simulink model "virtual_v11"  (R2022a)
settings: Solver=VariableStepAuto  StartTime=0.0  StopTime=50  RelTol=1e-3
libraries: slpidlib x5
settings Model: Creator=leona  LastModifiedBy=leona

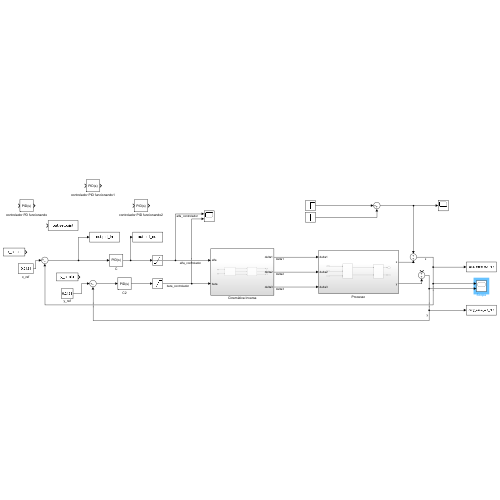
[thumbnail: Simulink's stored preview of the top-level diagram]
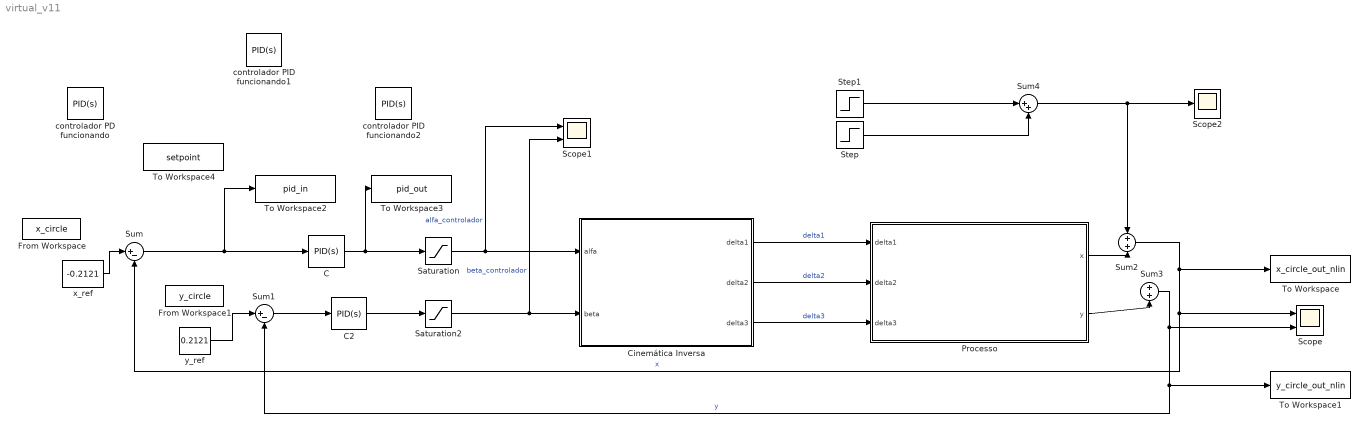
== system virtual_v11 ==
  C : slpidlib/PID Controller  Controller=PID  Form=Parallel  TimeDomain=Continuous-time  UseExternalTs=off  SampleTime=-1  IntegratorMethod=Forward Euler  FilterMethod=Forward Euler  ControllerParametersSource=internal  P=-0.3  I=-0.05  UseKiTs=off  D=-0.45  N=100  UseFilter=on  TunerSelectOption=Transfer Function Based (PID Tuner App)  InitialConditionSource=internal  InitialConditionForIntegrator=0  InitialConditionForFilter=0  DifferentiatorICPrevScaledInput=0  ExternalReset=none  TrackingMode=off  Kt=1  LimitOutput=off  SatLimitsSource=internal  UpperSaturationLimit=inf  LowerSaturationLimit=-inf  LinearizeAsGain=on  AntiWindupMode=none  Kb=1  POutMin=[]  POutMax=[]  IOutMin=[]  IOutMax=[]  DOutMin=[]  DOutMax=[]  NOutMin=[]  NOutMax=[]  SumOutMin=[]  SumOutMax=[]  SaturationOutMin=[]  SaturationOutMax=[]  PParamMin=[]  PParamMax=[]  IParamMin=[]  IParamMax=[]  DParamMin=[]  DParamMax=[]  NParamMin=[]  NParamMax=[]  KbParamMin=[]  KbParamMax=[]  KtParamMin=[]  KtParamMax=[]  KbOutMin=[]  KbOutMax=[]  KtOutMin=[]  KtOutMax=[]  IntegratorOutMin=[]  IntegratorOutMax=[]  FilterOutMin=[]  FilterOutMax=[]  SumI1OutMin=[]  SumI1OutMax=[]  SumI2OutMin=[]  SumI2OutMax=[]  SumI3OutMin=[]  SumI3OutMax=[]  SumI4OutMin=[]  SumI4OutMax=[]  SumDOutMin=[]  SumDOutMax=[]  DifferentiatorOutMin=[]  DifferentiatorOutMax=[]  FilterDiffOutCoefMin=[]  FilterDiffOutCoefMax=[]  ReciprocalOutMin=[]  ReciprocalOutMax=[]  SumDenOutMin=[]  SumDenOutMax=[]  SumNumOutMin=[]  SumNumOutMax=[]  DivideOutMin=[]  DivideOutMax=[]  UdiffTsProdOutMin=[]  UdiffTsProdOutMax=[]  NTsProdOutMin=[]  NTsProdOutMax=[]  UintegralTsProdOutMin=[]  UintegralTsProdOutMax=[]  UngainTsProdOutMin=[]  UngainTsProdOutMax=[]  IntegratorContinuousStateAttributes=''  IntegratorStateMustResolveToSignalObject=off  IntegratorRTWStateStorageClass=Auto  FilterContinuousStateAttributes=''  FilterStateMustResolveToSignalObject=off  FilterRTWStateStorageClass=Auto  ParallelPVariant=InternalParameters  IdealPVariant=Disabled  IVariant=InternalParameters  DVariant=InternalParameters  IntegratorVariant=Continuous  SatVariant=Disabled  AWVariant=Passthrough  PCopyVariant=Disabled  TRVariant=Disabled  FdbkBlocksVariant=Forward  IdealPFdbkVariant=Disabled  SatFdbkVariant=Disabled  DerivativeFilterVariant=ContFilter  NVariant=InternalParameters  NCopyVariant=Disabled  FilterICVariant=InternalICsFilter  IntegratorICVariant=InternalICs  ExternalResetVariant=Disabled  TRSumVariant=Passthrough  SumFdbkVariant=Disabled  SumVariant=Sum_PID  TsampFilterVariant=InternalTs  TsampNgainVariant=Passthrough  TsampIntegralVariant=Passthrough  ExternalSaturationOutDataTypeStr=Inherit: Same as second input  aMode=0
  C2 : slpidlib/PID Controller  Controller=PID  Form=Parallel  TimeDomain=Continuous-time  UseExternalTs=off  SampleTime=-1  IntegratorMethod=Forward Euler  FilterMethod=Forward Euler  ControllerParametersSource=internal  P=-0.3  I=-0.05  UseKiTs=off  D=-0.45  N=100  UseFilter=on  TunerSelectOption=Transfer Function Based (PID Tuner App)  InitialConditionSource=internal  InitialConditionForIntegrator=0  InitialConditionForFilter=0  DifferentiatorICPrevScaledInput=0  ExternalReset=none  TrackingMode=off  Kt=1  LimitOutput=off  SatLimitsSource=internal  UpperSaturationLimit=inf  LowerSaturationLimit=-inf  LinearizeAsGain=on  AntiWindupMode=none  Kb=1  POutMin=[]  POutMax=[]  IOutMin=[]  IOutMax=[]  DOutMin=[]  DOutMax=[]  NOutMin=[]  NOutMax=[]  SumOutMin=[]  SumOutMax=[]  SaturationOutMin=[]  SaturationOutMax=[]  PParamMin=[]  PParamMax=[]  IParamMin=[]  IParamMax=[]  DParamMin=[]  DParamMax=[]  NParamMin=[]  NParamMax=[]  KbParamMin=[]  KbParamMax=[]  KtParamMin=[]  KtParamMax=[]  KbOutMin=[]  KbOutMax=[]  KtOutMin=[]  KtOutMax=[]  IntegratorOutMin=[]  IntegratorOutMax=[]  FilterOutMin=[]  FilterOutMax=[]  SumI1OutMin=[]  SumI1OutMax=[]  SumI2OutMin=[]  SumI2OutMax=[]  SumI3OutMin=[]  SumI3OutMax=[]  SumI4OutMin=[]  SumI4OutMax=[]  SumDOutMin=[]  SumDOutMax=[]  DifferentiatorOutMin=[]  DifferentiatorOutMax=[]  FilterDiffOutCoefMin=[]  FilterDiffOutCoefMax=[]  ReciprocalOutMin=[]  ReciprocalOutMax=[]  SumDenOutMin=[]  SumDenOutMax=[]  SumNumOutMin=[]  SumNumOutMax=[]  DivideOutMin=[]  DivideOutMax=[]  UdiffTsProdOutMin=[]  UdiffTsProdOutMax=[]  NTsProdOutMin=[]  NTsProdOutMax=[]  UintegralTsProdOutMin=[]  UintegralTsProdOutMax=[]  UngainTsProdOutMin=[]  UngainTsProdOutMax=[]  IntegratorContinuousStateAttributes=''  IntegratorStateMustResolveToSignalObject=off  IntegratorRTWStateStorageClass=Auto  FilterContinuousStateAttributes=''  FilterStateMustResolveToSignalObject=off  FilterRTWStateStorageClass=Auto  ParallelPVariant=InternalParameters  IdealPVariant=Disabled  IVariant=InternalParameters  DVariant=InternalParameters  IntegratorVariant=Continuous  SatVariant=Disabled  AWVariant=Passthrough  PCopyVariant=Disabled  TRVariant=Disabled  FdbkBlocksVariant=Forward  IdealPFdbkVariant=Disabled  SatFdbkVariant=Disabled  DerivativeFilterVariant=ContFilter  NVariant=InternalParameters  NCopyVariant=Disabled  FilterICVariant=InternalICsFilter  IntegratorICVariant=InternalICs  ExternalResetVariant=Disabled  TRSumVariant=Passthrough  SumFdbkVariant=Disabled  SumVariant=Sum_PID  TsampFilterVariant=InternalTs  TsampNgainVariant=Passthrough  TsampIntegralVariant=Passthrough  ExternalSaturationOutDataTypeStr=Inherit: Same as second input  aMode=0
  Cinemática Inversa : Subsystem
  From Workspace : FromWorkspace  VariableName=x_circle
  From Workspace1 : FromWorkspace  VariableName=y_circle
  Processo : Subsystem
  Saturation : Saturate  UpperLimit=10  LowerLimit=-10
  Saturation2 : Saturate  UpperLimit=10  LowerLimit=-10
  Scope : Scope  NumInputPorts=2
  Scope1 : Scope  NumInputPorts=2
  Scope2 : Scope
  Step : Step  Time=40  After=-0.01  SampleTime=0
  Step1 : Step  Time=39  After=0.01  SampleTime=0
  Sum : Sum  Inputs=|+-
  Sum1 : Sum  Inputs=|+-
  Sum2 : Sum  Inputs=+|+
  Sum3 : Sum  Inputs=+|+
  Sum4 : Sum  Inputs=|++
  To Workspace : ToWorkspace  VariableName=x_circle_out_nlin  SaveFormat=Timeseries  SampleTime=-1
  To Workspace1 : ToWorkspace  VariableName=y_circle_out_nlin  SaveFormat=Timeseries  SampleTime=-1
  To Workspace2 : ToWorkspace  VariableName=pid_in  SaveFormat=Timeseries  SampleTime=-1
  To Workspace3 : ToWorkspace  VariableName=pid_out  SaveFormat=Timeseries  SampleTime=-1
  To Workspace4 : ToWorkspace  VariableName=setpoint  SaveFormat=Timeseries  SampleTime=-1
  controlador PD funcionando : slpidlib/PID Controller  Controller=PID  Form=Parallel  TimeDomain=Continuous-time  UseExternalTs=off  SampleTime=-1  IntegratorMethod=Forward Euler  FilterMethod=Forward Euler  ControllerParametersSource=internal  P=-0.3  I=0  UseKiTs=off  D=-0.337  N=100  UseFilter=on  TunerSelectOption=Transfer Function Based (PID Tuner App)  InitialConditionSource=internal  InitialConditionForIntegrator=0  InitialConditionForFilter=0  DifferentiatorICPrevScaledInput=0  ExternalReset=none  TrackingMode=off  Kt=1  LimitOutput=off  SatLimitsSource=internal  UpperSaturationLimit=inf  LowerSaturationLimit=-inf  LinearizeAsGain=on  AntiWindupMode=none  Kb=1  POutMin=[]  POutMax=[]  IOutMin=[]  IOutMax=[]  DOutMin=[]  DOutMax=[]  NOutMin=[]  NOutMax=[]  SumOutMin=[]  SumOutMax=[]  SaturationOutMin=[]  SaturationOutMax=[]  PParamMin=[]  PParamMax=[]  IParamMin=[]  IParamMax=[]  DParamMin=[]  DParamMax=[]  NParamMin=[]  NParamMax=[]  KbParamMin=[]  KbParamMax=[]  KtParamMin=[]  KtParamMax=[]  KbOutMin=[]  KbOutMax=[]  KtOutMin=[]  KtOutMax=[]  IntegratorOutMin=[]  IntegratorOutMax=[]  FilterOutMin=[]  FilterOutMax=[]  SumI1OutMin=[]  SumI1OutMax=[]  SumI2OutMin=[]  SumI2OutMax=[]  SumI3OutMin=[]  SumI3OutMax=[]  SumI4OutMin=[]  SumI4OutMax=[]  SumDOutMin=[]  SumDOutMax=[]  DifferentiatorOutMin=[]  DifferentiatorOutMax=[]  FilterDiffOutCoefMin=[]  FilterDiffOutCoefMax=[]  ReciprocalOutMin=[]  ReciprocalOutMax=[]  SumDenOutMin=[]  SumDenOutMax=[]  SumNumOutMin=[]  SumNumOutMax=[]  DivideOutMin=[]  DivideOutMax=[]  UdiffTsProdOutMin=[]  UdiffTsProdOutMax=[]  NTsProdOutMin=[]  NTsProdOutMax=[]  UintegralTsProdOutMin=[]  UintegralTsProdOutMax=[]  UngainTsProdOutMin=[]  UngainTsProdOutMax=[]  IntegratorContinuousStateAttributes=''  IntegratorStateMustResolveToSignalObject=off  IntegratorRTWStateStorageClass=Auto  FilterContinuousStateAttributes=''  FilterStateMustResolveToSignalObject=off  FilterRTWStateStorageClass=Auto  ParallelPVariant=InternalParameters  IdealPVariant=Disabled  IVariant=InternalParameters  DVariant=InternalParameters  IntegratorVariant=Continuous  SatVariant=Disabled  AWVariant=Passthrough  PCopyVariant=Disabled  TRVariant=Disabled  FdbkBlocksVariant=Forward  IdealPFdbkVariant=Disabled  SatFdbkVariant=Disabled  DerivativeFilterVariant=ContFilter  NVariant=InternalParameters  NCopyVariant=Disabled  FilterICVariant=InternalICsFilter  IntegratorICVariant=InternalICs  ExternalResetVariant=Disabled  TRSumVariant=Passthrough  SumFdbkVariant=Disabled  SumVariant=Sum_PID  TsampFilterVariant=InternalTs  TsampNgainVariant=Passthrough  TsampIntegralVariant=Passthrough  ExternalSaturationOutDataTypeStr=Inherit: Same as second input  aMode=0
  controlador PID funcionando1 : slpidlib/PID Controller  Controller=PID  Form=Parallel  TimeDomain=Continuous-time  UseExternalTs=off  SampleTime=-1  IntegratorMethod=Forward Euler  FilterMethod=Forward Euler  ControllerParametersSource=internal  P=-0.032597  I=-0.0018862  UseKiTs=off  D=-0.14083  N=100  UseFilter=on  TunerSelectOption=Transfer Function Based (PID Tuner App)  InitialConditionSource=internal  InitialConditionForIntegrator=0  InitialConditionForFilter=0  DifferentiatorICPrevScaledInput=0  ExternalReset=none  TrackingMode=off  Kt=1  LimitOutput=off  SatLimitsSource=internal  UpperSaturationLimit=inf  LowerSaturationLimit=-inf  LinearizeAsGain=on  AntiWindupMode=none  Kb=1  POutMin=[]  POutMax=[]  IOutMin=[]  IOutMax=[]  DOutMin=[]  DOutMax=[]  NOutMin=[]  NOutMax=[]  SumOutMin=[]  SumOutMax=[]  SaturationOutMin=[]  SaturationOutMax=[]  PParamMin=[]  PParamMax=[]  IParamMin=[]  IParamMax=[]  DParamMin=[]  DParamMax=[]  NParamMin=[]  NParamMax=[]  KbParamMin=[]  KbParamMax=[]  KtParamMin=[]  KtParamMax=[]  KbOutMin=[]  KbOutMax=[]  KtOutMin=[]  KtOutMax=[]  IntegratorOutMin=[]  IntegratorOutMax=[]  FilterOutMin=[]  FilterOutMax=[]  SumI1OutMin=[]  SumI1OutMax=[]  SumI2OutMin=[]  SumI2OutMax=[]  SumI3OutMin=[]  SumI3OutMax=[]  SumI4OutMin=[]  SumI4OutMax=[]  SumDOutMin=[]  SumDOutMax=[]  DifferentiatorOutMin=[]  DifferentiatorOutMax=[]  FilterDiffOutCoefMin=[]  FilterDiffOutCoefMax=[]  ReciprocalOutMin=[]  ReciprocalOutMax=[]  SumDenOutMin=[]  SumDenOutMax=[]  SumNumOutMin=[]  SumNumOutMax=[]  DivideOutMin=[]  DivideOutMax=[]  UdiffTsProdOutMin=[]  UdiffTsProdOutMax=[]  NTsProdOutMin=[]  NTsProdOutMax=[]  UintegralTsProdOutMin=[]  UintegralTsProdOutMax=[]  UngainTsProdOutMin=[]  UngainTsProdOutMax=[]  IntegratorContinuousStateAttributes=''  IntegratorStateMustResolveToSignalObject=off  IntegratorRTWStateStorageClass=Auto  FilterContinuousStateAttributes=''  FilterStateMustResolveToSignalObject=off  FilterRTWStateStorageClass=Auto  ParallelPVariant=InternalParameters  IdealPVariant=Disabled  IVariant=InternalParameters  DVariant=InternalParameters  IntegratorVariant=Continuous  SatVariant=Disabled  AWVariant=Passthrough  PCopyVariant=Disabled  TRVariant=Disabled  FdbkBlocksVariant=Forward  IdealPFdbkVariant=Disabled  SatFdbkVariant=Disabled  DerivativeFilterVariant=ContFilter  NVariant=InternalParameters  NCopyVariant=Disabled  FilterICVariant=InternalICsFilter  IntegratorICVariant=InternalICs  ExternalResetVariant=Disabled  TRSumVariant=Passthrough  SumFdbkVariant=Disabled  SumVariant=Sum_PID  TsampFilterVariant=InternalTs  TsampNgainVariant=Passthrough  TsampIntegralVariant=Passthrough  ExternalSaturationOutDataTypeStr=Inherit: Same as second input  aMode=0
  controlador PID funcionando2 : slpidlib/PID Controller  Controller=PID  Form=Parallel  TimeDomain=Continuous-time  UseExternalTs=off  SampleTime=-1  IntegratorMethod=Forward Euler  FilterMethod=Forward Euler  ControllerParametersSource=internal  P=-0.30287  I=-0.051401  UseKiTs=off  D=-0.44616  N=100  UseFilter=on  TunerSelectOption=Transfer Function Based (PID Tuner App)  InitialConditionSource=internal  InitialConditionForIntegrator=0  InitialConditionForFilter=0  DifferentiatorICPrevScaledInput=0  ExternalReset=none  TrackingMode=off  Kt=1  LimitOutput=off  SatLimitsSource=internal  UpperSaturationLimit=inf  LowerSaturationLimit=-inf  LinearizeAsGain=on  AntiWindupMode=none  Kb=1  POutMin=[]  POutMax=[]  IOutMin=[]  IOutMax=[]  DOutMin=[]  DOutMax=[]  NOutMin=[]  NOutMax=[]  SumOutMin=[]  SumOutMax=[]  SaturationOutMin=[]  SaturationOutMax=[]  PParamMin=[]  PParamMax=[]  IParamMin=[]  IParamMax=[]  DParamMin=[]  DParamMax=[]  NParamMin=[]  NParamMax=[]  KbParamMin=[]  KbParamMax=[]  KtParamMin=[]  KtParamMax=[]  KbOutMin=[]  KbOutMax=[]  KtOutMin=[]  KtOutMax=[]  IntegratorOutMin=[]  IntegratorOutMax=[]  FilterOutMin=[]  FilterOutMax=[]  SumI1OutMin=[]  SumI1OutMax=[]  SumI2OutMin=[]  SumI2OutMax=[]  SumI3OutMin=[]  SumI3OutMax=[]  SumI4OutMin=[]  SumI4OutMax=[]  SumDOutMin=[]  SumDOutMax=[]  DifferentiatorOutMin=[]  DifferentiatorOutMax=[]  FilterDiffOutCoefMin=[]  FilterDiffOutCoefMax=[]  ReciprocalOutMin=[]  ReciprocalOutMax=[]  SumDenOutMin=[]  SumDenOutMax=[]  SumNumOutMin=[]  SumNumOutMax=[]  DivideOutMin=[]  DivideOutMax=[]  UdiffTsProdOutMin=[]  UdiffTsProdOutMax=[]  NTsProdOutMin=[]  NTsProdOutMax=[]  UintegralTsProdOutMin=[]  UintegralTsProdOutMax=[]  UngainTsProdOutMin=[]  UngainTsProdOutMax=[]  IntegratorContinuousStateAttributes=''  IntegratorStateMustResolveToSignalObject=off  IntegratorRTWStateStorageClass=Auto  FilterContinuousStateAttributes=''  FilterStateMustResolveToSignalObject=off  FilterRTWStateStorageClass=Auto  ParallelPVariant=InternalParameters  IdealPVariant=Disabled  IVariant=InternalParameters  DVariant=InternalParameters  IntegratorVariant=Continuous  SatVariant=Disabled  AWVariant=Passthrough  PCopyVariant=Disabled  TRVariant=Disabled  FdbkBlocksVariant=Forward  IdealPFdbkVariant=Disabled  SatFdbkVariant=Disabled  DerivativeFilterVariant=ContFilter  NVariant=InternalParameters  NCopyVariant=Disabled  FilterICVariant=InternalICsFilter  IntegratorICVariant=InternalICs  ExternalResetVariant=Disabled  TRSumVariant=Passthrough  SumFdbkVariant=Disabled  SumVariant=Sum_PID  TsampFilterVariant=InternalTs  TsampNgainVariant=Passthrough  TsampIntegralVariant=Passthrough  ExternalSaturationOutDataTypeStr=Inherit: Same as second input  aMode=0
  x_ref : Constant  Value=-0.2121
  y_ref : Constant  Value=0.2121
  wires:
  Cinemática Inversa/1(delta1) -> Processo/1(delta1)  "delta1"
  Cinemática Inversa/2(delta2) -> Processo/2(delta2)  "delta2"
  Cinemática Inversa/3(delta3) -> Processo/3(delta3)  "delta3"
  Saturation/1 -> Scope1/1, Cinemática Inversa/1(alfa)  "alfa_controlador"
  Saturation2/1 -> Scope1/2, Cinemática Inversa/2(beta)  "beta_controlador"
  C/1 -> To Workspace3/1, Saturation/1
  Processo/2(y) -> Sum3/2
  Processo/1(x) -> Sum2/2
  Sum2/1 -> Scope/1, Sum/2, To Workspace/1  "x"
  Sum3/1 -> To Workspace1/1, Sum1/2, Scope/2  "y"
  C2/1 -> Saturation2/1
  Sum/1 -> C/1, To Workspace2/1
  Sum1/1 -> C2/1
  Sum4/1 -> Sum2/1, Scope2/1
  Step1/1 -> Sum4/1
  Step/1 -> Sum4/2
  x_ref/1 -> Sum/1
  y_ref/1 -> Sum1/1

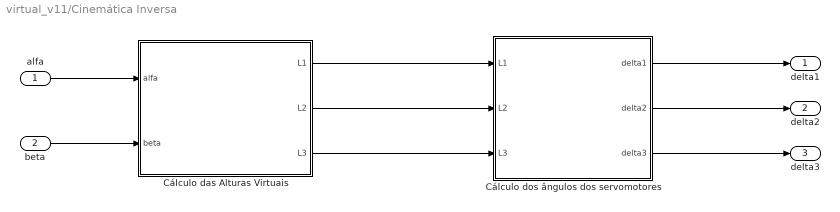
== system virtual_v11/Cinemática Inversa ==
  alfa : Inport
  beta : Inport  Port=2
  Cálculo das Alturas Virtuais : Subsystem
  Cálculo dos ângulos dos servomotores : Subsystem
  delta1 : Outport
  delta2 : Outport  Port=2
  delta3 : Outport  Port=3
  wires:
  alfa/1 -> Cálculo das Alturas Virtuais/1(alfa)
  beta/1 -> Cálculo das Alturas Virtuais/2(beta)
  Cálculo das Alturas Virtuais/1(L1) -> Cálculo dos ângulos dos servomotores/1(L1)
  Cálculo das Alturas Virtuais/2(L2) -> Cálculo dos ângulos dos servomotores/2(L2)
  Cálculo das Alturas Virtuais/3(L3) -> Cálculo dos ângulos dos servomotores/3(L3)
  Cálculo dos ângulos dos servomotores/1(delta1) -> delta1/1
  Cálculo dos ângulos dos servomotores/2(delta2) -> delta2/1
  Cálculo dos ângulos dos servomotores/3(delta3) -> delta3/1

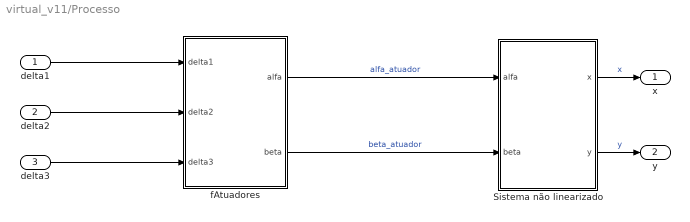
== system virtual_v11/Processo ==
  delta1 : Inport
  delta2 : Inport  Port=2
  delta3 : Inport  Port=3
  Sistema não linearizado : Subsystem
  fAtuadores : MATLAB Function  TreatAsAtomicUnit=on
  x : Outport
  y : Outport  Port=2
  wires:
  fAtuadores/2(beta) -> Sistema não linearizado/2(beta)  "beta_atuador"
  delta3/1 -> fAtuadores/3(delta3)
  delta2/1 -> fAtuadores/2(delta2)
  delta1/1 -> fAtuadores/1(delta1)
  Sistema não linearizado/2(y) -> y/1  "y"
  Sistema não linearizado/1(x) -> x/1  "x"
  fAtuadores/1(alfa) -> Sistema não linearizado/1(alfa)  "alfa_atuador"

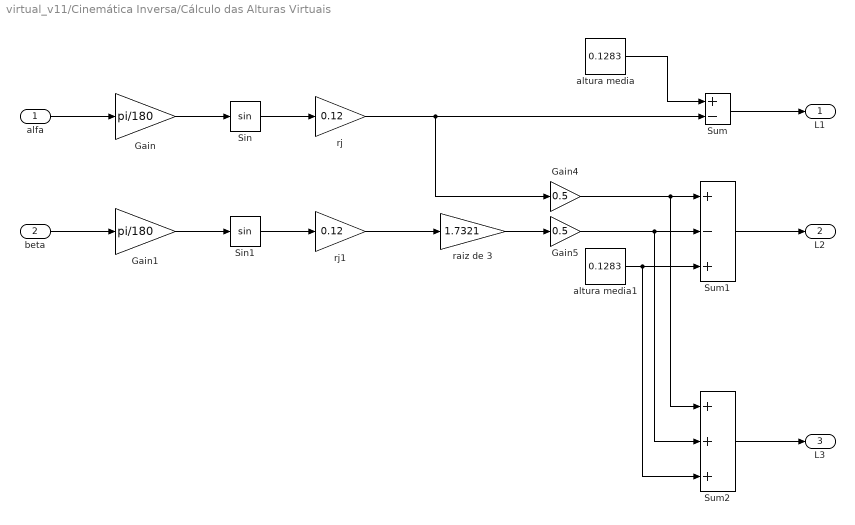
== system virtual_v11/Cinemática Inversa/Cálculo das Alturas Virtuais ==
  alfa : Inport
  beta : Inport  Port=2
  Gain : Gain  Gain=pi/180
  Gain1 : Gain  Gain=pi/180
  Gain4 : Gain  Gain=0.5
  Gain5 : Gain  Gain=0.5
  Sin : Trigonometry
  Sin1 : Trigonometry
  Sum : Sum  Inputs=+-
  Sum1 : Sum  Inputs=+-+
  Sum2 : Sum  Inputs=+++
  altura media : Constant  Value=0.1283
  altura media1 : Constant  Value=0.1283
  raiz de 3 : Gain  Gain=1.7321
  rj : Gain  Gain=0.12
  rj1 : Gain  Gain=0.12
  L1 : Outport
  L2 : Outport  Port=2
  L3 : Outport  Port=3
  wires:
  alfa/1 -> Gain/1
  beta/1 -> Gain1/1
  Gain/1 -> Sin/1
  Gain1/1 -> Sin1/1
  Sum/1 -> L1/1
  altura media/1 -> Sum/1
  Sin/1 -> rj/1
  rj/1 -> Gain4/1, Sum/2
  Sin1/1 -> rj1/1
  Sum1/1 -> L2/1
  Gain4/1 -> Sum2/1, Sum1/1
  raiz de 3/1 -> Gain5/1
  rj1/1 -> raiz de 3/1
  altura media1/1 -> Sum2/3, Sum1/3
  Sum2/1 -> L3/1
  Gain5/1 -> Sum2/2, Sum1/2

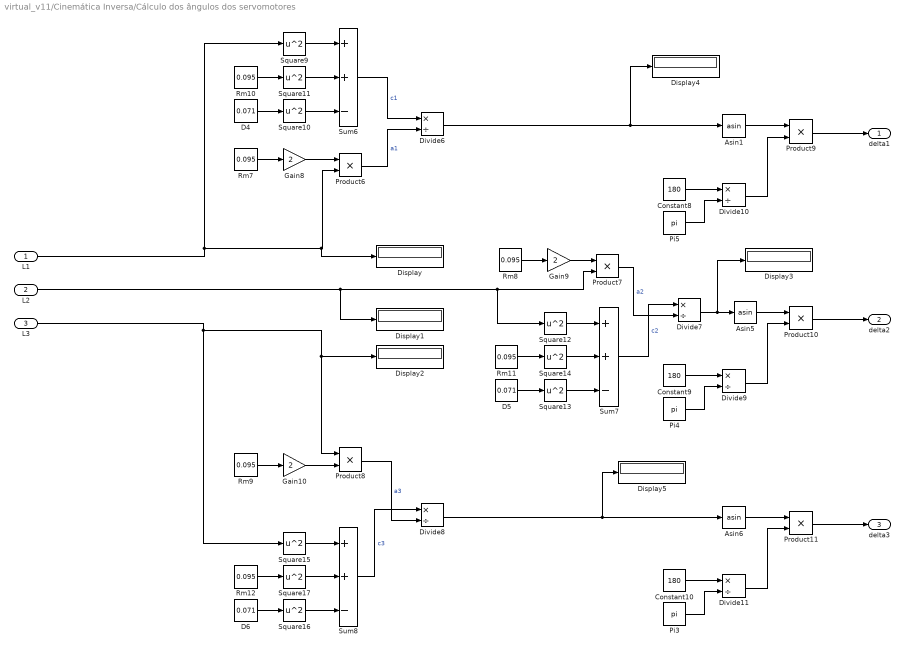
== system virtual_v11/Cinemática Inversa/Cálculo dos ângulos dos servomotores ==
  L1 : Inport
  L2 : Inport  Port=2
  L3 : Inport  Port=3
  Asin1 : Trigonometry  Operator=asin
  Asin5 : Trigonometry  Operator=asin
  Asin6 : Trigonometry  Operator=asin
  Constant10 : Constant  Value=180
  Constant8 : Constant  Value=180
  Constant9 : Constant  Value=180
  D4 : Constant  Value=0.071
  D5 : Constant  Value=0.071
  D6 : Constant  Value=0.071
  Display{,1..5} (6 alike) : Display
  Divide{6..11} (6 alike) : Product  Inputs=*/
  Gain10 : Gain  Gain=2
  Gain8 : Gain  Gain=2
  Gain9 : Gain  Gain=2
  Pi3 : Constant  Value=pi  OutDataTypeStr=Inherit: Inherit via back propagation
  Pi4 : Constant  Value=pi  OutDataTypeStr=Inherit: Inherit via back propagation
  Pi5 : Constant  Value=pi  OutDataTypeStr=Inherit: Inherit via back propagation
  Product{6..11} (6 alike) : Product
  Rm{7..12} (6 alike) : Constant  Value=0.095
  Square{9..17} (9 alike) : Math  Operator=square
  Sum6 : Sum  Inputs=++-
  Sum7 : Sum  Inputs=++-
  Sum8 : Sum  Inputs=++-
  delta1 : Outport
  delta2 : Outport  Port=2
  delta3 : Outport  Port=3
  wires:
  Divide10/1 -> Product9/2
  Square13/1 -> Sum7/3
  Constant9/1 -> Divide9/1
  Rm7/1 -> Gain8/1
  L1/1 -> Square9/1, Display/1, Product6/2
  Pi3/1 -> Divide11/2
  Square16/1 -> Sum8/3
  D5/1 -> Square13/1
  Asin6/1 -> Product11/1
  Pi5/1 -> Divide10/2
  Divide11/1 -> Product11/2
  Square17/1 -> Sum8/2
  Asin1/1 -> Product9/1
  Constant10/1 -> Divide11/1
  Gain8/1 -> Product6/1
  Rm8/1 -> Gain9/1
  Sum7/1 -> Divide7/1  "c2"
  Square15/1 -> Sum8/1
  L2/1 -> Display1/1, Square12/1, Product7/2
  Gain9/1 -> Product7/1
  Product6/1 -> Divide6/2  "a1"
  Product8/1 -> Divide8/2  "a3"
  Square12/1 -> Sum7/1
  Rm11/1 -> Square14/1
  Square9/1 -> Sum6/1
  Rm10/1 -> Square11/1
  Rm12/1 -> Square17/1
  Product10/1 -> delta2/1
  Divide6/1 -> Display4/1, Asin1/1
  Divide8/1 -> Display5/1, Asin6/1
  Divide7/1 -> Display3/1, Asin5/1
  Pi4/1 -> Divide9/2
  D6/1 -> Square16/1
  Constant8/1 -> Divide10/1
  Sum6/1 -> Divide6/1  "c1"
  Gain10/1 -> Product8/2
  L3/1 -> Square15/1, Display2/1, Product8/1
  Product7/1 -> Divide7/2  "a2"
  Sum8/1 -> Divide8/1  "c3"
  Rm9/1 -> Gain10/1
  Square10/1 -> Sum6/3
  Square14/1 -> Sum7/2
  Asin5/1 -> Product10/1
  Square11/1 -> Sum6/2
  Divide9/1 -> Product10/2
  D4/1 -> Square10/1
  Product11/1 -> delta3/1
  Product9/1 -> delta1/1

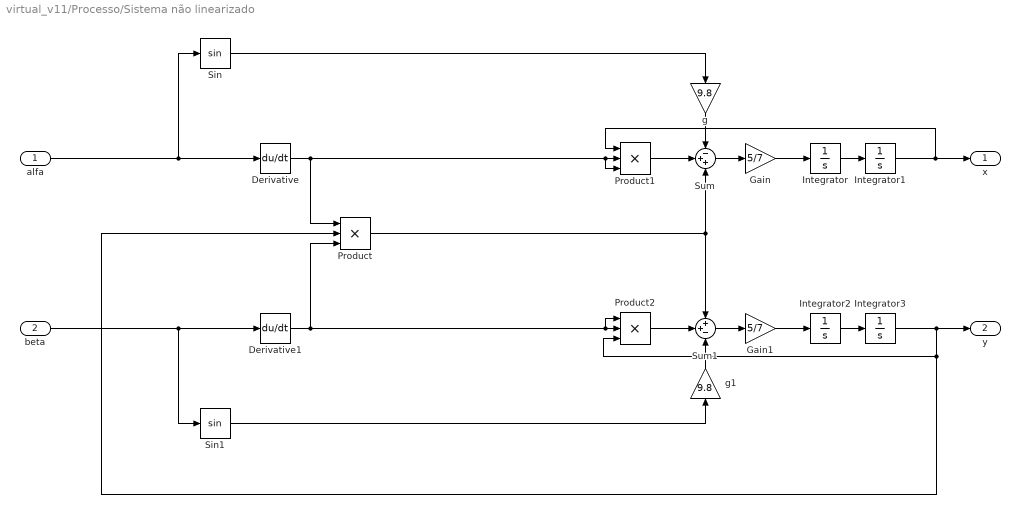
== system virtual_v11/Processo/Sistema não linearizado ==
  alfa : Inport
  beta : Inport  Port=2
  Derivative : Derivative
  Derivative1 : Derivative
  Gain : Gain  Gain=5/7
  Gain1 : Gain  Gain=5/7
  Integrator{,1..3} (4 alike) : Integrator
  Product : Product  Inputs=3
  Product1 : Product  Inputs=3
  Product2 : Product  Inputs=3
  Sin : Trigonometry
  Sin1 : Trigonometry
  Sum : Sum  Inputs=-++
  Sum1 : Sum  Inputs=++-
  g : Gain  Gain=9.8
  g1 : Gain  Gain=9.8
  x : Outport
  y : Outport  Port=2
  wires:
  Integrator/1 -> Integrator1/1
  Integrator1/1 -> Product1/1, x/1
  Integrator2/1 -> Integrator3/1
  Gain/1 -> Integrator/1
  Gain1/1 -> Integrator2/1
  Sum1/1 -> Gain1/1
  Sum/1 -> Gain/1
  g1/1 -> Sum1/3
  Sin1/1 -> g1/1
  alfa/1 -> Derivative/1, Sin/1
  beta/1 -> Derivative1/1, Sin1/1
  g/1 -> Sum/1
  Sin/1 -> g/1
  Derivative1/1 -> Product2/1, Product2/2, Product/3
  Derivative/1 -> Product1/3, Product1/2, Product/1
  Integrator3/1 -> Product/2, Product2/3, y/1
  Product2/1 -> Sum1/2
  Product1/1 -> Sum/2
  Product/1 -> Sum1/1, Sum/3

== matlab function virtual_v11/Processo/fAtuadores ==
  data: delta1 input; alfa output; delta2 input; delta3 input; beta output
function [alfa, beta] = atuadores(delta1, delta2, delta3)

rj = 0.12;
%rm = 0.11;
% Rm = 0.071;
% D = 0.095;
Rm = 0.071;
D = 0.095;
h = 0.145;

alfa = 0;
beta = 0;

inic = [0 0 0];
delta = inic + [delta1, delta2, delta3];
delta = deg2rad(delta);

l1 = Rm*sin(delta(1)) - sqrt(D^2 - cos(delta(1))^2*Rm^2);
if l1 < 0
    l1 = Rm*sin(delta(1)) + sqrt(D^2 - cos(delta(1))^2*Rm^2);
end

l2 = Rm*sin(delta(2)) - sqrt(D^2 - cos(delta(2))^2*Rm^2);
if l2 < 0
    l2 = Rm*sin(delta(2)) + sqrt(D^2 - cos(delta(2))^2*Rm^2);
end

l3 = Rm*sin(delta(3)) - sqrt(D^2 - cos(delta(3))^2*Rm^2);
if l3 < 0
    l3 = Rm*sin(delta(3)) + sqrt(D^2 - cos(delta(3))^2*Rm^2);
end

L = [l1 l2 l3];

beta = asin((L(3)-L(2))/(rj*sqrt(3)));
beta = rad2deg(beta);

alfa = asin((L(2)+L(3)-2*L(1))/(3*rj));
alfa = rad2deg(alfa);

end
